simulink model "linear_model"  (R2017a)
settings: Solver=VariableStepAuto  StartTime=0.0  StopTime=10.0  RelTol=1e-3
undefined symbols (not defined in the file): Discrete, Time
libraries: dspstat3 x2, ctrlSharedLib x1
settings Model: Creator=Achierius  LastModifiedBy=Achierius

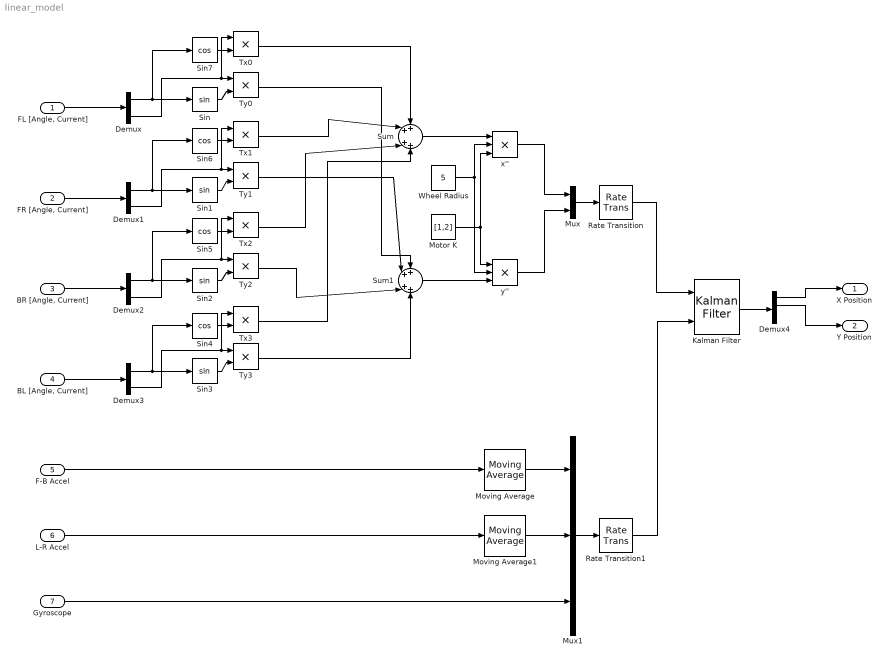
== system linear_model ==
  "FL [Angle, Current]" : Inport
  "FR [Angle, Current]" : Inport  Port=2
  "BR [Angle, Current]" : Inport  Port=3
  "BL [Angle, Current]" : Inport  Port=4
  F-B Accel : Inport  Port=5
  L-R Accel : Inport  Port=6
  Gyroscope : Inport  Port=7
  Demux{,1..3} (4 alike) : Demux  Outputs=2
  Demux4 : Demux  Outputs=6
  Kalman Filter : ctrlSharedLib/Kalman Filter  TimeDomain=Discrete-Time  UseCurrentEstimator=on  ModelSource=Individual A, B, C, D matrices  ModelSourceVariable=ss(0.95,1,1,0,1)  A=[[1,0.002,0,0,0,0],[0,1,0,0,0,0],[0,0,1,0.002,0,0],[0,0,0,1,0,0],[0,0,0,0,1,0.002],[0,0,0,0,0,1]]  B=[[2e-6,0],[0.002,0],[0,2e-6],[0,0.002],[0,0],[0,0]]  C=[[0,0,0,0,0,0],[0,0,0,0,0,0],[0,0,0,0,0,1]]  D=0  NumberOfStates=6  NumberOfInputs=2  NumberOfOutputs=2  InitialEstimateSource=Dialog  X0=0  P0=10  UseK=off  UseGH=off  NumberOfProcessNoiseInputs=1  G=1  TimeInvariantG=on  H=0  TimeInvariantH=on  Q=0.05  TimeInvariantQ=on  R=1  TimeInvariantR=on  N=0  TimeInvariantN=on  AddInputPort=on  AddEnablePort=off  OutputEstimatedY=off  OutputP=off  Ts=-1
  Motor K : Constant  Value=[1,2]
  Moving Average : dspstat3/Moving Average  Method=Sliding window  SpecifyWindowLength=on  WindowLength=4  ForgettingFactor=0.9  SimulateUsing=Code generation
  Moving Average1 : dspstat3/Moving Average  Method=Sliding window  SpecifyWindowLength=on  WindowLength=4  ForgettingFactor=0.9  SimulateUsing=Code generation
  Mux : Mux  Inputs=2
  Mux1 : Mux  Inputs=3
  Rate Transition : RateTransition  OutPortSampleTime=[0.002,0]
  Rate Transition1 : RateTransition  OutPortSampleTime=[0.002,0]
  Sin{,1..3} (4 alike) : Trigonometry
  Sin{4..7} (4 alike) : Trigonometry  Operator=cos
  Sum : Sum  Inputs=++|++
  Sum1 : Sum  Inputs=++|++
  Tx{0..3} (4 alike) : Product
  Ty{0..3} (4 alike) : Product
  Wheel Radius : Constant  Value=5
  x'' : Product  Inputs=3
  y'' : Product  Inputs=3
  X Position : Outport
  Y Position : Outport  Port=2
  wires:
  F-B Accel/1 -> Moving Average/1
  "BR [Angle, Current]"/1 -> Demux2/1
  Sin1/1 -> Ty1/2
  "FR [Angle, Current]"/1 -> Demux1/1
  Mux1/1 -> Rate Transition1/1
  Demux2/1 -> Sin5/1, Sin2/1
  Sin6/1 -> Tx1/2
  Tx1/1 -> Sum/2
  Demux2/2 -> Tx2/1, Ty2/1
  Sin2/1 -> Ty2/2
  Sin4/1 -> Tx3/2
  Ty0/1 -> Sum1/1
  L-R Accel/1 -> Moving Average1/1
  Demux4/3 -> Y Position/1
  Motor K/1 -> x''/3, y''/1
  "FL [Angle, Current]"/1 -> Demux/1
  x''/1 -> Mux/1
  Rate Transition/1 -> Kalman Filter/1
  Demux3/1 -> Sin4/1, Sin3/1
  Sin3/1 -> Ty3/2
  Sum/1 -> x''/1
  Wheel Radius/1 -> y''/2, x''/2
  Gyroscope/1 -> Mux1/3
  Demux1/1 -> Sin6/1, Sin1/1
  Moving Average1/1 -> Mux1/2
  Kalman Filter/1 -> Demux4/1
  Demux/1 -> Sin7/1, Sin/1
  Demux1/2 -> Tx1/1, Ty1/1
  Tx3/1 -> Sum/4
  Mux/1 -> Rate Transition/1
  Ty3/1 -> Sum1/4
  "BL [Angle, Current]"/1 -> Demux3/1
  Demux3/2 -> Tx3/1, Ty3/1
  Demux/2 -> Tx0/1, Ty0/1
  Ty2/1 -> Sum1/3
  y''/1 -> Mux/2
  Sin/1 -> Ty0/2
  Ty1/1 -> Sum1/2
  Rate Transition1/1 -> Kalman Filter/2
  Tx2/1 -> Sum/3
  Moving Average/1 -> Mux1/1
  Sum1/1 -> y''/3
  Sin5/1 -> Tx2/2
  Tx0/1 -> Sum/1
  Demux4/1 -> X Position/1
  Sin7/1 -> Tx0/2
